simulink model "sim_hcw_nmpc"  (R2022b)
settings: Solver=ode45  StartTime=0.0  StopTime=tfin  FixedStep=1  RelTol=1e-3  EnableMultiTasking=on
values from neighbouring files (symbols this model uses):
  K = nmpc_design_st(par)    [main_hcw_nmpc.m]
  r = [5 0 0 0 0 0]'    [main_hcw_nmpc.m]
undefined symbols (not defined in the file or in its folder): nlcon
libraries: cstblocks x1
settings Model: Creator=carlonovara  LastModifiedBy=Enf
settings SolverCC: AlgebraicLoopSolver=TrustRegion  AutoInsertRateTranBlk=on
settings DataIOCC: ReturnWorkspaceOutputs=off
settings OptimizationCC: LifeSpan=inf
settings DebuggingCC: UnconnectedInputMsg=warning  UnconnectedOutputMsg=warning  UnconnectedLineMsg=warning  SFUnexpectedBacktrackingDiag=warning  SFNoUnconditionalDefaultTransitionDiag=warning  SFExecutionAtInitializationDiag=none  SFMachineParentedDataDiag=warning  ArithmeticOperatorsInVariantConditions=warning
settings HardwareCC: ProdBitPerSizeT=32  ProdBitPerPtrDiffT=32  ProdWordSize=32  ProdHWDeviceType=Specified
settings ModelReferenceCC: EnableRefExpFcnMdlSchedulingChecks=on
settings SFSimCC: SimUseLocalCustomCode=off  CustomCodeUndefinedFunction=UseInterfaceOnly
settings RTWCC: RTWUseLocalCustomCode=off  DLArmComputeVersion=19.05
settings CodeAppCC: StateflowObjectComments=on
settings GRTTargetCC: TargetLangStandard=C89/C90 (ANSI)
settings ConfigComp: CovMetricSettings=dw  CovSaveCumulativeToWorkspaceVar=on  CovSaveSingleToWorkspaceVar=on  CovExternalEMLEnable=off

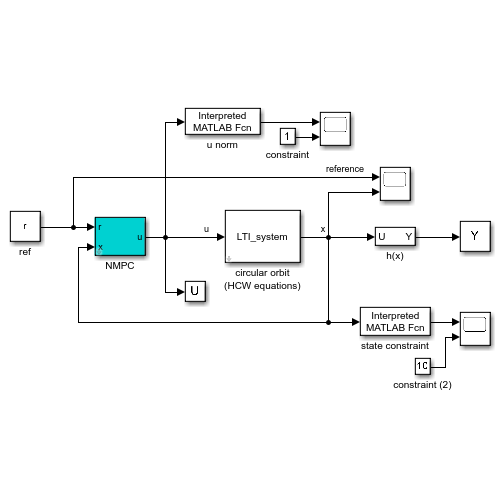
[thumbnail: Simulink's stored preview of the top-level diagram]
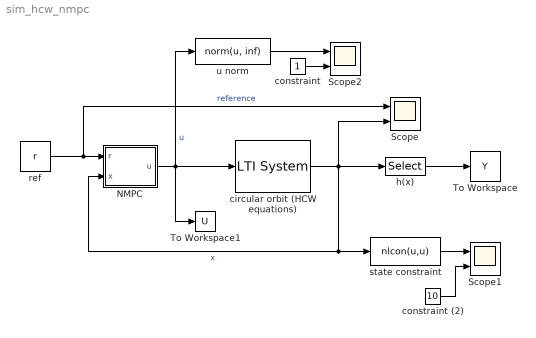
== system sim_hcw_nmpc ==
  NMPC : Subsystem  mask{K=K}
      mask prompts: K "NMPC structure"
  Scope : Scope  NumInputPorts=2
  Scope1 : Scope  NumInputPorts=2
  Scope2 : Scope  NumInputPorts=2
  To Workspace : ToWorkspace  VariableName=Y  SaveFormat=Timeseries  SampleTime=-1
  To Workspace1 : ToWorkspace  VariableName=U  SaveFormat=Timeseries  SampleTime=-1
  circular orbit (HCW equations) : cstblocks/LTI System  sys=LTI_system  IC=x0
  constraint : Constant
  constraint (2) : Constant  Value=10
  h(x) : Selector  InputPortWidth=6  IndexOptions=Index vector (dialog)  Indices=1:3  OutputSizes=1
  ref : Constant  Value=r  SampleTime=-1
  state constraint : MATLABFcn  MATLABFcn=nlcon(u,u)
  u norm : MATLABFcn  MATLABFcn=norm(u, inf)
  wires:
  circular orbit (HCW equations)/1 -> NMPC/2(x), state constraint/1, h(x)/1, Scope/2  "x"
  state constraint/1 -> Scope1/1
  NMPC/1(u) -> u norm/1, circular orbit (HCW equations)/1, To Workspace1/1  "u"
  ref/1 -> Scope/1, NMPC/1(r)  "reference"
  h(x)/1 -> To Workspace/1
  constraint/1 -> Scope2/2
  u norm/1 -> Scope2/1
  constraint (2)/1 -> Scope1/2

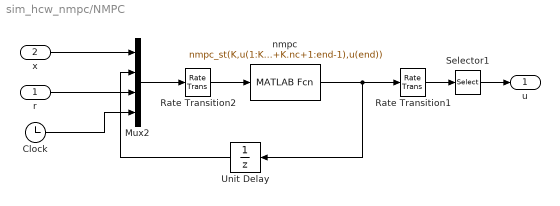
== system sim_hcw_nmpc/NMPC ==
  r : Inport
  x : Inport  Port=2
  Clock : Clock
  Mux2 : Mux
  Rate Transition1 : RateTransition  OutPortSampleTime=K.Ts
  Rate Transition2 : RateTransition  OutPortSampleTime=K.Ts
  Selector1 : Selector  InputPortWidth=K.nc  IndexOptions=Index vector (dialog)  Indices=1:K.nu  OutputSizes=1
  Unit Delay : UnitDelay  InitialCondition=zeros(K.nc,1)  SampleTime=K.Ts  HasFrameUpgradeWarning=on
  nmpc : MATLABFcn  MATLABFcn=nmpc_st(K,u(1:K.nx),u(K.nx+1:K.nx+K.nc),u(K.nx+K.nc+1:end-1),u(end))  OutputDimensions=K.nc
  u : Outport
  wires:
  Selector1/1 -> u/1
  Unit Delay/1 -> Mux2/2
  nmpc/1 -> Unit Delay/1, Rate Transition1/1
  Rate Transition1/1 -> Selector1/1
  Mux2/1 -> Rate Transition2/1
  x/1 -> Mux2/1
  r/1 -> Mux2/3
  Clock/1 -> Mux2/4
  Rate Transition2/1 -> nmpc/1
